simulink model "btp_VERSION2_draft1"  (R2020a)
settings: Solver=VariableStepAuto  StartTime=0.0  StopTime=1e5  RelTol=1e-3
PreLoadFcn:
  | building_length = 15; % m
  | building_width = 10; % m
  | building_height = 2.5; % m
  | 
  | wall_thickness = 0.2; % m
  | wall_density = 2000; % kg/m^3
  | wall_specific_heat = 840; % J/(kg*K)
  | wall_conductivity = 0.04; % W/(m*K)
  | wall_heat_transfer_coeff_internal = 25; % W/(m^2*K)
  | wall_heat_transfer_coeff_external = 35; % W/(m^2*K)
  | 
  | roof_thickness = 0.2; % m
  | roof_density = 2000; % kg/m^3
  | roof_specific_heat = 840; % J/(kg*K)
  | roof_conductivity = 0.035; % W/(m*K)
  | roof_heat_transfer_coeff_internal = 10; % W/(m^2*K)
  | roof_heat_transfer_coeff_external = 30; % W/(m^2*K)
  | 
  | floor_thickness = 0.1; % m
  | floor_conductivity = 0.15; % W/(m*K)
  | floor_heat_transfer_coeff_internal = 15; % W/(m^2*K)
  | 
  | door_area = 2*0.6; % m^2
  | 
  | duct_area = 0.1^2; % m^2
  | 
  | fan_setting_table = 0 : 4; % 1
  | fan_flow_rate_table = [0 0.08 0.12 0.16 0.2]; % kg/s
  | 
  | initial_temperature = 35; % degC
  | ground_temperature = 25; % degC
  | 
  | flow_reversal_Mach = 1e-5; % 1
InitFcn:
  | zone_volume = building_length * building_width * building_height / 4; % m^3
  | zone_flow_area = 0.7 * building_height * (building_length + building_width) / 4; % m^2
model workspace (MAT data in the model file):
  CO2_occupant = 0.01
  N_occupant = 1
  T_occupant = 30
  W_occupant = 70
  y_co2_env = 0.04
undefined symbols (not defined in the file): mdot_coolant, sigbuilder_block, T_coolant
libraries: fl_lib x57, nesl_utility x23, HVAC_lib x1
(part 2 of 2)

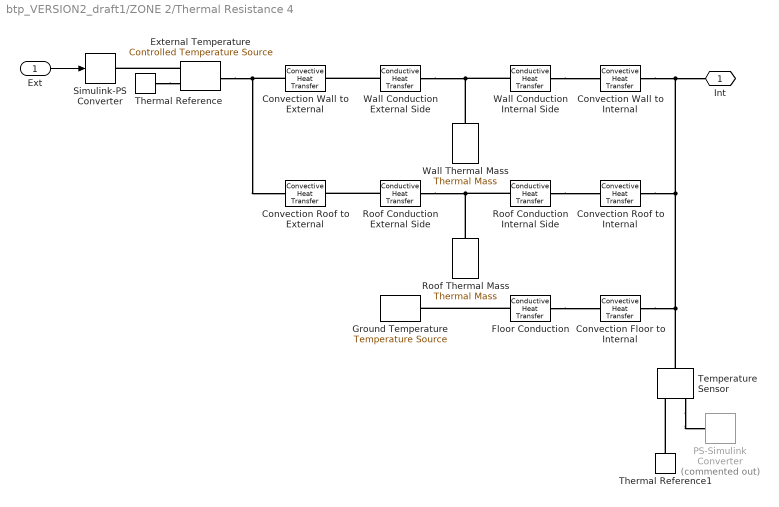
== system btp_VERSION2_draft1/ZONE 2/Thermal Resistance 4 ==
  Ext : Inport
  Convection Floor to Internal : fl_lib/Thermal/Thermal Elements/Convective Heat Transfer  area=floor_area m^2  heat_tr_coeff=floor_heat_transfer_coeff_internal W/(m^2 * K)  T_specify=off  T_priority=None  T=0 K  T_nominal_specify=off  T_nominal_unit=K  T_nominal_value=1  Q_specify=off  Q_priority=None  Q=0 W  Q_nominal_specify=off  Q_nominal_unit=W  Q_nominal_value=1
  Convection Roof to External : fl_lib/Thermal/Thermal Elements/Convective Heat Transfer  area=roof_area m^2  heat_tr_coeff=roof_heat_transfer_coeff_external W/(m^2 * K)  T_specify=off  T_priority=None  T=0 K  T_nominal_specify=off  T_nominal_unit=K  T_nominal_value=1  Q_specify=off  Q_priority=None  Q=0 W  Q_nominal_specify=off  Q_nominal_unit=W  Q_nominal_value=1
  Convection Roof to Internal : fl_lib/Thermal/Thermal Elements/Convective Heat Transfer  area=roof_area m^2  heat_tr_coeff=roof_heat_transfer_coeff_internal W/(m^2 * K)  T_specify=off  T_priority=None  T=0 K  T_nominal_specify=off  T_nominal_unit=K  T_nominal_value=1  Q_specify=off  Q_priority=None  Q=0 W  Q_nominal_specify=off  Q_nominal_unit=W  Q_nominal_value=1
  Convection Wall to External : fl_lib/Thermal/Thermal Elements/Convective Heat Transfer  area=wall_area m^2  heat_tr_coeff=wall_heat_transfer_coeff_external W/(m^2 * K)  T_specify=off  T_priority=None  T=0 K  T_nominal_specify=off  T_nominal_unit=K  T_nominal_value=1  Q_specify=off  Q_priority=None  Q=0 W  Q_nominal_specify=off  Q_nominal_unit=W  Q_nominal_value=1
  Convection Wall to Internal : fl_lib/Thermal/Thermal Elements/Convective Heat Transfer  area=wall_area m^2  heat_tr_coeff=wall_heat_transfer_coeff_internal W/(m^2 * K)  T_specify=off  T_priority=None  T=0 K  T_nominal_specify=off  T_nominal_unit=K  T_nominal_value=1  Q_specify=off  Q_priority=None  Q=0 W  Q_nominal_specify=off  Q_nominal_unit=W  Q_nominal_value=1
  External Temperature : fl_lib/Thermal/Thermal Sources/Controlled Temperature Source
  Floor Conduction : fl_lib/Thermal/Thermal Elements/Conductive Heat Transfer  area=floor_area m^2  thickness=floor_thickness m  th_cond=floor_conductivity W/(m*K)  T_specify=off  T_priority=None  T=0 K  T_nominal_specify=off  T_nominal_unit=K  T_nominal_value=1  Q_specify=off  Q_priority=None  Q=0 W  Q_nominal_specify=off  Q_nominal_unit=W  Q_nominal_value=1
  Ground Temperature : fl_lib/Thermal/Thermal Sources/Temperature Source  temperature=ground_temperature degC
  PS-Simulink Converter : nesl_utility/PS-Simulink Converter  Commented=on  PhysicalDomain=network_engine_domain  SubClassName=ps_output  LeftPortType=input  RightPortType=output  PseudoPeriodic=off  Frequencies=[]  Unit=degC  AffineConversion=on
  Roof Conduction External Side : fl_lib/Thermal/Thermal Elements/Conductive Heat Transfer  area=roof_area m^2  thickness=roof_thickness / 2 m  th_cond=roof_conductivity W/(m*K)  T_specify=off  T_priority=None  T=0 K  T_nominal_specify=off  T_nominal_unit=K  T_nominal_value=1  Q_specify=off  Q_priority=None  Q=0 W  Q_nominal_specify=off  Q_nominal_unit=W  Q_nominal_value=1
  Roof Conduction Internal Side : fl_lib/Thermal/Thermal Elements/Conductive Heat Transfer  area=roof_area m^2  thickness=roof_thickness / 2 m  th_cond=roof_conductivity W/(m*K)  T_specify=off  T_priority=None  T=0 K  T_nominal_specify=off  T_nominal_unit=K  T_nominal_value=1  Q_specify=off  Q_priority=None  Q=0 W  Q_nominal_specify=off  Q_nominal_unit=W  Q_nominal_value=1
  Roof Thermal Mass : fl_lib/Thermal/Thermal Elements/Thermal Mass  mass=roof_area * roof_thickness * wall_density kg  sp_heat=roof_specific_heat J/kg/K  T_specify=on  T_priority=High  T=roof_initial_temperature degC  T_nominal_specify=off  T_nominal_unit=K  T_nominal_value=1  Q_specify=off  Q_priority=None  Q=0 W  Q_nominal_specify=off  Q_nominal_unit=W  Q_nominal_value=1
  Simulink-PS Converter : nesl_utility/Simulink-PS Converter  PhysicalDomain=network_engine_domain  SubClassName=ps_input  LeftPortType=input  RightPortType=output  PseudoPeriodic=off  Frequencies=[]  NoiseDistribution=none  NoiseParameters=[]  Unit=degC  AffineConversion=on  FilteringAndDerivatives=provide  SimscapeFilterOrder=1  InputFilterTimeConstant=0.001  UdotUserProvided=0
  Temperature Sensor : fl_lib/Thermal/Thermal Sensors/Temperature Sensor
  Thermal Reference : fl_lib/Thermal/Thermal Elements/Thermal Reference
  Thermal Reference1 : fl_lib/Thermal/Thermal Elements/Thermal Reference
  Wall Conduction External Side : fl_lib/Thermal/Thermal Elements/Conductive Heat Transfer  area=wall_area m^2  thickness=wall_thickness / 2 m  th_cond=wall_conductivity W/(m*K)  T_specify=off  T_priority=None  T=0 K  T_nominal_specify=off  T_nominal_unit=K  T_nominal_value=1  Q_specify=off  Q_priority=None  Q=0 W  Q_nominal_specify=off  Q_nominal_unit=W  Q_nominal_value=1
  Wall Conduction Internal Side : fl_lib/Thermal/Thermal Elements/Conductive Heat Transfer  area=wall_area m^2  thickness=wall_thickness / 2 m  th_cond=wall_conductivity W/(m*K)  T_specify=off  T_priority=None  T=0 K  T_nominal_specify=off  T_nominal_unit=K  T_nominal_value=1  Q_specify=off  Q_priority=None  Q=0 W  Q_nominal_specify=off  Q_nominal_unit=W  Q_nominal_value=1
  Wall Thermal Mass : fl_lib/Thermal/Thermal Elements/Thermal Mass  mass=wall_area * wall_thickness * wall_density kg  sp_heat=wall_specific_heat J/kg/K  T_specify=on  T_priority=High  T=wall_initial_temperature degC  T_nominal_specify=off  T_nominal_unit=K  T_nominal_value=1  Q_specify=off  Q_priority=None  Q=0 W  Q_nominal_specify=off  Q_nominal_unit=W  Q_nominal_value=1
  Int : PMIOPort  Side=Right
  wires:
  Ext/1 -> Simulink-PS Converter/1
  connections:
  Thermal Reference/LConn1 -- External Temperature/RConn2
  Temperature Sensor/RConn2 -- PS-Simulink Converter/LConn1
  Thermal Reference1/LConn1 -- Temperature Sensor/RConn1
  Floor Conduction/LConn1 -- Ground Temperature/LConn1
  Floor Conduction/RConn1 -- Convection Floor to Internal/LConn1
  Roof Conduction Internal Side/RConn1 -- Convection Roof to Internal/LConn1
  Roof Conduction External Side/LConn1 -- Convection Roof to External/RConn1
  Roof Conduction Internal Side/LConn1 -- Roof Thermal Mass/LConn1 -- Roof Conduction External Side/RConn1
  Wall Conduction Internal Side/LConn1 -- Wall Thermal Mass/LConn1 -- Wall Conduction External Side/RConn1
  Wall Conduction External Side/LConn1 -- Convection Wall to External/RConn1
  Convection Wall to External/LConn1 -- Convection Roof to External/LConn1 -- External Temperature/LConn1
  Convection Floor to Internal/RConn1 -- Int/RConn1 -- Convection Wall to Internal/RConn1 -- Convection Roof to Internal/RConn1 -- Temperature Sensor/LConn1
  Wall Conduction Internal Side/RConn1 -- Convection Wall to Internal/LConn1
  External Temperature/RConn1 -- Simulink-PS Converter/RConn1
